simulink model "PHY_AdaptiveMod_AryaMGC"  (R2024b)
settings: Solver=FixedStepAuto  StartTime=0.0  StopTime=35  FixedStep=1  RelTol=1e-3
settings Model: Creator=ARYA MGC  LastModifiedBy=ARYA MGC

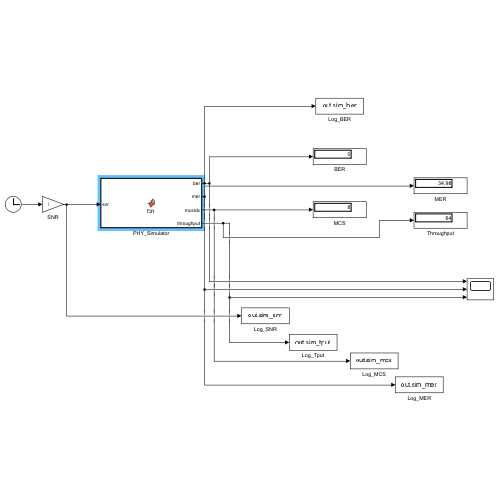
[thumbnail: Simulink's stored preview of the top-level diagram]
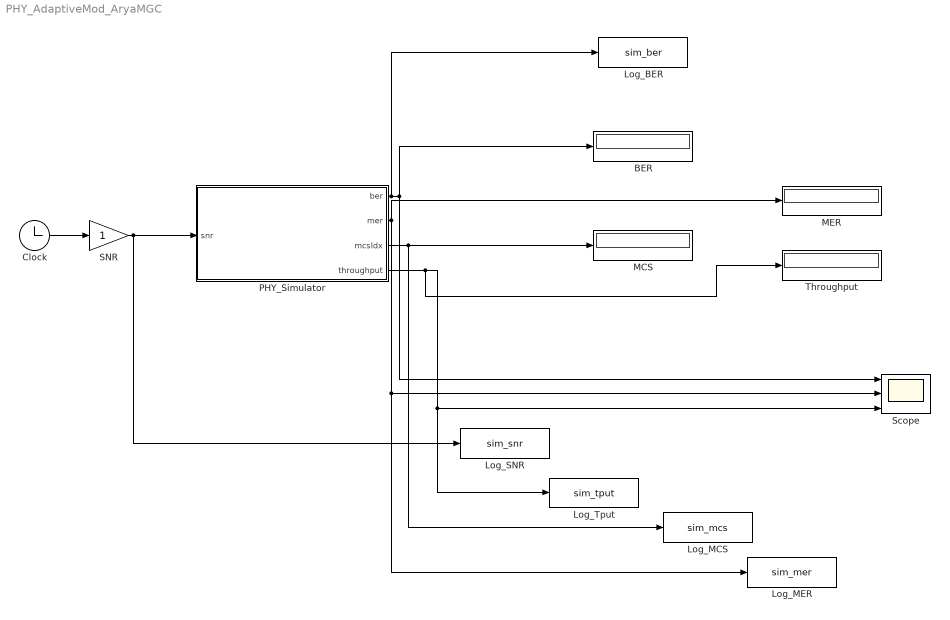
== system PHY_AdaptiveMod_AryaMGC ==
  BER : Display
  Clock : Clock
  Log_BER : ToWorkspace  VariableName=sim_ber  SampleTime=-1
  Log_MCS : ToWorkspace  VariableName=sim_mcs  SampleTime=-1
  Log_MER : ToWorkspace  VariableName=sim_mer  SampleTime=-1
  Log_SNR : ToWorkspace  VariableName=sim_snr  SampleTime=-1
  Log_Tput : ToWorkspace  VariableName=sim_tput  SampleTime=-1
  MCS : Display
  MER : Display
  PHY_Simulator : MATLAB Function  TreatAsAtomicUnit=on
  SNR : Gain
  Scope : Scope  NumInputPorts=3
  Throughput : Display
  wires:
  Clock/1 -> SNR/1
  SNR/1 -> PHY_Simulator/1(snr), Log_SNR/1
  PHY_Simulator/1(ber) -> BER/1, Scope/1, Log_BER/1
  PHY_Simulator/2(mer) -> Log_MER/1, Scope/2, MER/1
  PHY_Simulator/3(mcsIdx) -> Log_MCS/1, MCS/1
  PHY_Simulator/4(throughput) -> Log_Tput/1, Scope/3, Throughput/1

== matlab function PHY_AdaptiveMod_AryaMGC/PHY_Simulator ==
  data: snr input; ber output; mer output; mcsIdx output; throughput output
function [ber, mer, mcsIdx, throughput] = fcn(snr)
coder.extrinsic('run_phy_step');
if snr >= 28
    modOrder = 256; bps = 8; mcsIdx = 8;
elseif snr >= 24
    modOrder = 64; bps = 6; mcsIdx = 7;
elseif snr >= 20
    modOrder = 64; bps = 6; mcsIdx = 6;
elseif snr >= 16
    modOrder = 16; bps = 4; mcsIdx = 5;
elseif snr >= 12
    modOrder = 16; bps = 4; mcsIdx = 4;
elseif snr >= 9
    modOrder = 4; bps = 2; mcsIdx = 3;
elseif snr >= 5
    modOrder = 4; bps = 2; mcsIdx = 2;
else
    modOrder = 2; bps = 1; mcsIdx = 1;
end

ber = double(0); mer = double(0); throughput = double(0);
[ber, mer, throughput] = run_phy_step(snr, modOrder, bps);
